simulink library "Latcher"  (R2019b)
settings: Solver=VariableStepAuto  StartTime=0.0  StopTime=10.0  RelTol=1e-3
settings Model: Creator=hp  LastModifiedBy=mehran

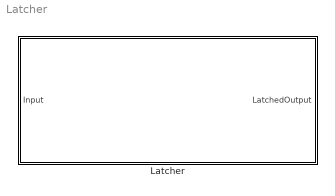
== system Latcher ==
  Latcher : Subsystem

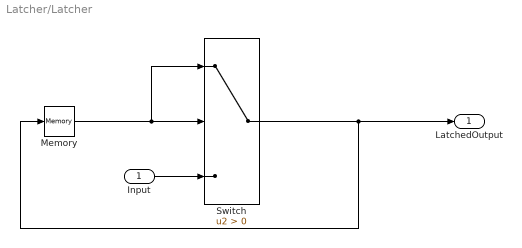
== system Latcher/Latcher ==
  Input : Inport
  Memory : Memory
  Switch : Switch  Criteria=u2 > Threshold
  LatchedOutput : Outport
  wires:
  Memory/1 -> Switch/1, Switch/2
  Switch/1 -> LatchedOutput/1, Memory/1
  Input/1 -> Switch/3
